simulink model "clock_toggle"  (R2020a)
settings: Solver=VariableStepAuto  StartTime=0.0  StopTime=inf  RelTol=1e-3
libraries: simulink_extras x1
settings Model: Creator=F1  LastModifiedBy=F1

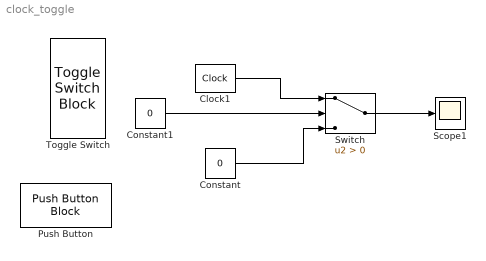
== system clock_toggle ==
  Clock1 : simulink_extras/Flip Flops/Clock  period=2
  Constant : Constant  Value=0
  Constant1 : Constant  Value=0
  Push Button : PushButtonBlock
  Scope1 : Scope
  Switch : Switch  Criteria=u2 > Threshold
  Toggle Switch : ToggleSwitchBlock
      settings: Values={{'Off', 'On'}, [0 1]}
  wires:
  Clock1/1 -> Switch/1
  Constant/1 -> Switch/3
  Constant1/1 -> Switch/2
  Switch/1 -> Scope1/1
